simulink model "equalizer_eml"  (Simulink 6.0)
settings: Solver=FixedStepDiscrete  SolverMode=SingleTasking  StartTime=0.0  StopTime=0.1  RelTol=1e-3
InitFcn:
  | equalizer_eml_init
values from neighbouring files (symbols this model uses):
  params = p    [wlan80211a_settings.m]
undefined symbols (not defined in the file or in its folder): qammod, slcm
libraries: commsink2 x4, dspsigattribs x4, commchan2 x2, commdigbbndam2 x2, dsparch4 x1, commrandsrc2 x1, dspsnks4 x1, simulink x1
CloseFcn:
  | clear params
  | clear logsOut
settings Model: CovMetricSettings=dmw  Creator=The Mathworks Inc.  LastModifiedBy=mclark  ExtModeAutoUpdateStatusClock=off
settings DataIOCC: LimitDataPoints=off  SaveOutput=off  SaveTime=off  SignalLoggingName=logsOut
settings OptimizationCC: InlineInvariantSignals=off  LifeSpan=1
settings DebuggingCC: CheckExecutionContextPreStartOutputMsg=on  CheckExecutionContextRuntimeOutputMsg=on  SolverPrmCheckMsg=none
settings HardwareCC: TargetUnknown=on
settings ModelReferenceCC: UpdateModelReferenceTargets=IfOutOfDate
settings RTWCC: SystemTargetFile=ert.tlc  TemplateMakefile=ert_default_tmf  GenerateReport=on  ProcessScript=ert_make_rtw_hook  LaunchReport=on
settings CodeAppCC: IgnoreCustomStorageClasses=off  MangleLength=5
settings ERTTargetCC: TargetFcnLib=ansi_tfl_tmw.mat  GenFloatMathFcnCalls=ANSI_C  GenerateSampleERTMain=on  SupportContinuousTime=on  SupportNonInlinedSFcns=on  RootIOFormat=Individual Arguments  ERTCustomFileTemplate=example_file_process.tlc  InitialValueSource=Model
settings SFSimCC: SFSimApplyToAllLibs=on  SFSimBuildMode=Incremental

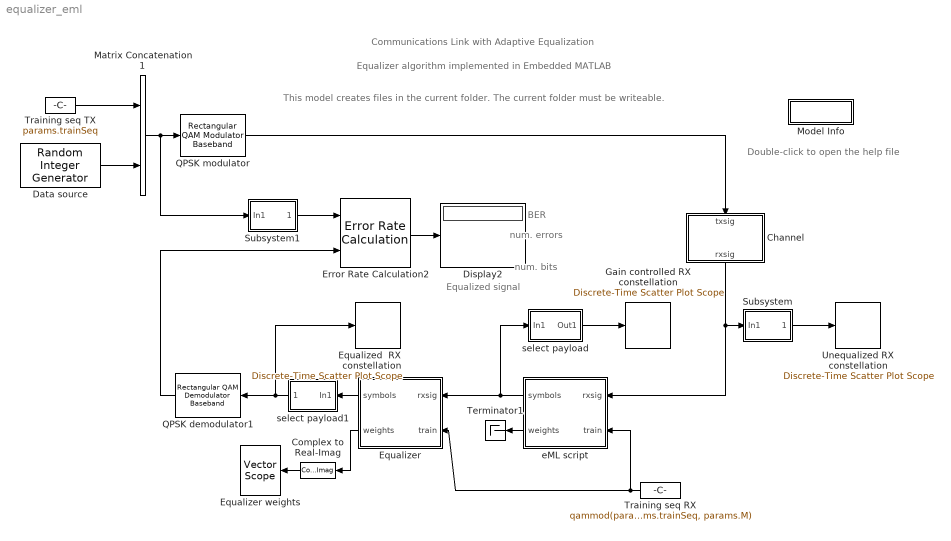
== system equalizer_eml ==
  note: Communications Link with Adaptive Equalization
  note: Equalizer algorithm implemented in Embedded MATLAB
  note: BER
  note: Equalized signal
  note: num. errors
  note: Double-click to open
      | the help file
  note: This model creates files in the current folder.
      | The current folder must be writeable.
  note: num. bits
  " Gain controlled RX constellation" : commsink2/Discrete-Time Scatter Plot Scope  Tag=ScatterPlot  sampPerSymb=1  offsetEye=0  numTraces=200  numNewFrames=100  LineMarkers=.  LineColors=b  fading=on  render=on  AxisGrid=on  xMin=-1.84900078842742  xMax=1.93655728027381  yMin=-1.87362349123512  yMax=1.91193457746611  inphaseLabel=In-phase Amplitude  quadratureLabel=Quadrature Amplitude  openScopeAtSimStart=on  FrameNumber=off  FigPos=[256 31 242 242]  figTitle=''  numLinesMax=8  block_type_=scatter
  Channel : Subsystem  Orientation=down  PropExecContextAcrossSSBoundary=on  mask(Multipath Rician fading chanel){gain_fade=[0 -9], gain_spec=[-10 -60], doppler=0.0001/params.symbolPeriod, SNRdB=60, T=params.symbolPeriod}
      mask prompts: gain_fade "Fading component gains (dB):"; gain_spec "Specular component gains (dB):"; doppler "Maximum Doppler shift (Hz):"; SNRdB "SNR (dB):"; T "Symbol period (s):"
      mask init:
      | gSpec = sum(10.^(gain_spec/10));
      | gFade = sum(10.^(gain_fade)/10);
      | gainChan = sqrt(0.5/(gSpec+gFade));
      | % factor of 0.5 for QPSK
      mask Display: disp('Rician Fading\nChannel')
  Complex to Real-Imag : ComplexToRealImag  Orientation=left  Output=Real
  Data source : commrandsrc2/Random Integer Generator  mul=4  seed=37  Ts=params.sourcePeriod  frameBased=on  sampPerFrame=params.Nsource  orient=off
  Display2 : Display
  Equalized  RX constellation : commsink2/Discrete-Time Scatter Plot Scope  Tag=ScatterPlot  sampPerSymb=1  offsetEye=0  numTraces=200  numNewFrames=100  LineMarkers=.  LineColors=b  fading=on  render=on  AxisGrid=on  xMin=-1.84900078842742  xMax=1.93655728027381  yMin=-1.87362349123512  yMax=1.91193457746611  inphaseLabel=In-phase Amplitude  quadratureLabel=Quadrature Amplitude  openScopeAtSimStart=on  FrameNumber=off  FigPos=[505 31 242 242]  figTitle=''  numLinesMax=8  block_type_=scatter
  Equalizer : Subsystem  Orientation=left  PropExecContextAcrossSSBoundary=on  mask(Receiver processing (adaptive equalizer)){eqMode=RLS, numWeights=6, refTap=4, resetWeights=off}
      mask prompts: eqMode "Adaptive algorithm:"; numWeights "Number of weights:"; refTap "Reference tap:"; resetWeights "Reset weights each frame"
      mask init:
      | if refTap<1 || refTap>numWeights
      | 	error(['Reference tap must be between 1 and ' num2str(numWeights)]);
      | end
      | stepSize = 0.025; % step size
      | lambda = 0.99; % forget factor
      | delta1 = 0.1 + 0i; % diagonal element of inv. corr. mtx.
      mask StyleString: popup(LMS|RLS),edit,edit,checkbox
  Equalizer weights : dspsnks4/Vector Scope  Orientation=left  ScopeProperties=off  Domain=User-defined  HorizSpan=1  DisplayProperties=off  AxisGrid=on  Memory=off  FrameNumber=off  AxisLegend=off  AxisZoom=off  OpenScopeAtSimStart=on  OpenScopeImmediately=off  FigPos=[756 30 251 243]  AxisProperties=off  XUnits=Hertz  XRange=[0...Fs/2]  InheritXIncr=off  XIncr=1  XLabel=delay  YUnits=dB  YLabel=Amplitude  LineProperties=off  LineMarkers=.  LineColors=[0 0 1]
      settings: YMin=-2  YMax=2
  Error Rate Calculation2 : commsink2/Error Rate Calculation  N=0  st_delay=0  cp_mode=Entire frame  subframe=[]  PMode=Port  WsName=ErrorVec  RsMode2=off  stop=off  numErr=100  maxBits=1e6
  Matrix Concatenation1 : simulink/Math Operations/Matrix Concatenation  numInports=2  catMethod=Vertical
  Model Info : Subsystem  LoadFcn=slcm LoadBlock;  InitFcn=slcm('UpdateAllCMBlocksInThisModelInit')  PropExecContextAcrossSSBoundary=on  mask(CMBlock){InitialSaveTempField=, InitialBlockCM=None, BlockCM=None, Frame=on, SaveTempField=, DisplayStringWithTags=Info, MaskDisplayString=Info, HorizontalTextAlignment=Center, LeftAlignmentValue=0.5, SourceBlockDiagram=equalizer_eml, TagMaxNumber=20, CMTag1=, CMTag2=, CMTag3=, CMTag4=, CMTag5=, CMTag6=, CMTag7=, CMTag8=, CMTag9=, CMTag10=, CMTag11=, CMTag12=, CMTag13=, CMTag14=, CMTag15=, CMTag16=, CMTag17=, CMTag18=, CMTag19=, CMTag20=}
      mask help: This block allows revision control information to be displayed within the model.
      settings: CopyFcn=slcm CopyBlock;  DeleteFcn=slcm Cancel;  PostSaveFcn=slcm('UpdateAllCMBlocksInThisModel')  NameChangeFcn=slcm Rename;  OpenFcn=commdemohelp;
      mask Display: text(str2num(LeftAlignmentValue), 0.5, MaskDisplayString, 'HorizontalAlignment', HorizontalTextAlignment)
  QPSK demodulator1 : commdigbbndam2/Rectangular QAM Demodulator Baseband  Orientation=left  M=params.M  OutType=Integer  Dec=Binary  PowType=Min. distance between symbols  MinDist=2  AvgPow=1  PeakPow=1  Ph=0  numSamp=1
  QPSK modulator : commdigbbndam2/Rectangular QAM Modulator Baseband  M=params.M  InType=Integer  Enc=Binary  PowType=Min. distance between symbols  MinDist=2  AvgPow=1  PeakPow=1  Ph=0  numSamp=1
  Subsystem : Subsystem  PropExecContextAcrossSSBoundary=on
      mask Display: disp('Select\nPayload')
  Subsystem1 : Subsystem  PropExecContextAcrossSSBoundary=on
      mask Display: disp('Select\nPayload')
  Terminator1 : Terminator
  Training seq RX : Constant  Orientation=left  Value=qammod(params.trainSeq, params.M)
  Training seq TX : Constant  Value=params.trainSeq
  Unequalized RX constellation : commsink2/Discrete-Time Scatter Plot Scope  Tag=ScatterPlot  sampPerSymb=1  offsetEye=0  numTraces=500  numNewFrames=50  LineMarkers=.  LineColors=b  fading=on  render=on  AxisGrid=on  xMin=-2  xMax=2  yMin=-2  yMax=2  inphaseLabel=In-phase Amplitude  quadratureLabel=Quadrature Amplitude  openScopeAtSimStart=on  FrameNumber=off  FigPos=[7 31 242 243]  figTitle=''  numLinesMax=8  block_type_=scatter
  eML script : Stateflow chart  Orientation=left  PropExecContextAcrossSSBoundary=on
  select payload : Subsystem  PropExecContextAcrossSSBoundary=on
      mask Display: disp('Select\nPayload')
  select payload1 : Subsystem  Orientation=left  PropExecContextAcrossSSBoundary=on
      mask Display: disp('Select\nPayload')
  wires:
  Subsystem/1(Out1) -> Unequalized RX constellation/1
  eML script/2(weights) -> Terminator1/1
  Training seq TX/1 -> Matrix Concatenation1/1
  Data source/1 -> Matrix Concatenation1/2
  Matrix Concatenation1/1 -> QPSK modulator/1, Subsystem1/1(In1)
  QPSK modulator/1 -> Channel/1(txsig)
  Subsystem1/1(Out1) -> Error Rate Calculation2/1
  Error Rate Calculation2/1 -> Display2/1
  eML script/1(symbols) -> select payload/1(In1), Equalizer/1(rxsig)
  select payload/1(Out1) -> " Gain controlled RX constellation"/1
  Channel/1(rxsig) -> eML script/1(rxsig), Subsystem/1(In1)
  Training seq RX/1 -> eML script/2(train), Equalizer/2(train)
  Equalizer/1(symbols) -> select payload1/1(In1)
  select payload1/1(Out1) -> QPSK demodulator1/1, Equalized  RX constellation/1
  QPSK demodulator1/1 -> Error Rate Calculation2/2
  Equalizer/2(weights) -> Complex to Real-Imag/1
  Complex to Real-Imag/1 -> Equalizer weights/1

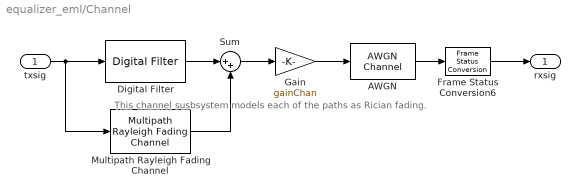
== system equalizer_eml/Channel ==
  note: This channel susbsystem models each
      | of the paths as Rician fading.
  txsig : Inport  LatchInput=off
  AWGN : commchan2/AWGN Channel  seed=67  noiseMode="Signal to noise ratio  (SNR)"  EbNodB=10  EsNodB=10  SNRdB=SNRdB  bitsPerSym=1  Ps=1  Tsym=1  variance=1
  Digital Filter : dsparch4/Digital Filter  DialogController=dspDDGCreate  DialogControllerArgs=DataTag0  TypePopup=FIR (all zeros)  IIRFiltStruct=Direct form II transposed  AllPoleFiltStruct=Direct form  FIRFiltStruct=Direct form  CoeffSource=Specify via dialog  NumCoeffs=10.^(gain_spec/20)  DenCoeffs=[1 0.1]  BiQuadCoeffs=[1 0.3 0.4 1 0.1 0.2]  LatticeCoeffs=[0.2 0.4]  denIgnore=on  FiltPerSampPopup=One filter per frame  IC=0  ICnum=0  ICden=0  roundingMode=Floor  overflowMode=off  ScaleValues=1  scaleValueFracLength=14  stageInFracLength=15  stageOutFracLength=15
  Frame Status Conversion6 : dspsigattribs/Frame Status Conversion  growRefPort=off  outframe=Sample-based
  Gain : Gain  Gain=gainChan  SaturateOnIntegerOverflow=on
  Multipath Rayleigh Fading Channel : commchan2/Multipath Rayleigh Fading Channel  Fd=doppler  simTs=T  delayVec=(0:length(gain_fade)-1)*T  gainVecdB=gain_fade  normGain=off  Seed=73
  Sum : Sum  Inputs=|++  SaturateOnIntegerOverflow=on
  rxsig : Outport
  wires:
  AWGN/1 -> Frame Status Conversion6/1
  txsig/1 -> Digital Filter/1, Multipath Rayleigh Fading Channel/1
  Sum/1 -> Gain/1
  Gain/1 -> AWGN/1
  Digital Filter/1 -> Sum/1
  Multipath Rayleigh Fading Channel/1 -> Sum/2
  Frame Status Conversion6/1 -> rxsig/1

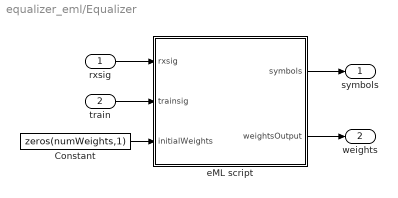
== system equalizer_eml/Equalizer ==
  rxsig : Inport  LatchInput=off
  train : Inport  Port=2  LatchInput=off
  Constant : Constant  Value=zeros(numWeights,1)  VectorParams1D=off
  eML script : Stateflow chart  PropExecContextAcrossSSBoundary=on
  symbols : Outport
  weights : Outport  Port=2
  wires:
  eML script/1(symbols) -> symbols/1
  eML script/2(weightsOutput) -> weights/1
  train/1 -> eML script/2(trainsig)
  rxsig/1 -> eML script/1(rxsig)
  Constant/1 -> eML script/3(initialWeights)

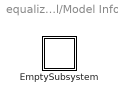
== system equalizer_eml/Model Info ==
  EmptySubsystem : Subsystem  PropExecContextAcrossSSBoundary=on

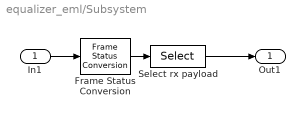
== system equalizer_eml/Subsystem ==
  In1 : Inport  LatchInput=off
  Frame Status Conversion : dspsigattribs/Frame Status Conversion  growRefPort=off  outframe=Frame-based
  Select rx payload : Selector  Elements=(params.Ntrain+1):(params.Nsymbols-10)  InputPortWidth=params.Nsymbols
  Out1 : Outport
  wires:
  In1/1 -> Frame Status Conversion/1
  Select rx payload/1 -> Out1/1
  Frame Status Conversion/1 -> Select rx payload/1

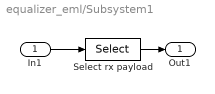
== system equalizer_eml/Subsystem1 ==
  In1 : Inport  LatchInput=off
  Select rx payload : Selector  Elements=(params.Ntrain+1):(params.Nsymbols-10)  InputPortWidth=params.Nsymbols
  Out1 : Outport
  wires:
  In1/1 -> Select rx payload/1
  Select rx payload/1 -> Out1/1

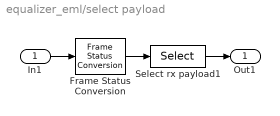
== system equalizer_eml/select payload ==
  In1 : Inport  LatchInput=off
  Frame Status Conversion : dspsigattribs/Frame Status Conversion  growRefPort=off  outframe=Frame-based
  Select rx payload1 : Selector  Elements=(params.Ntrain+1):(params.Nsymbols-10)  InputPortWidth=params.Nsymbols
  Out1 : Outport
  wires:
  Select rx payload1/1 -> Out1/1
  In1/1 -> Frame Status Conversion/1
  Frame Status Conversion/1 -> Select rx payload1/1

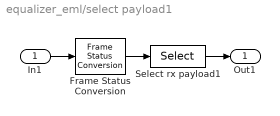
== system equalizer_eml/select payload1 ==
  In1 : Inport  LatchInput=off
  Frame Status Conversion : dspsigattribs/Frame Status Conversion  growRefPort=off  outframe=Frame-based
  Select rx payload1 : Selector  Elements=(params.Ntrain+1):(params.Nsymbols-10)  InputPortWidth=params.Nsymbols
  Out1 : Outport
  wires:
  Frame Status Conversion/1 -> Select rx payload1/1
  In1/1 -> Frame Status Conversion/1
  Select rx payload1/1 -> Out1/1

== system equalizer_eml/Model Info/EmptySubsystem ==

== matlab function eML script ==
  data: rxsig input double; train input double; symbols output double size=size(rxsig); weights output double
function [symbols, weights] = gaincontrol(rxsig, train)
% 1-tap adaptive equalizer using RLS algorithm

% Equalizer settings
lambda = 0.99; % forgetting factor for RLS

% Initialize
Delta = 0.1+0j; % inv. corr. parameter
weights = 0+0j;    

symbols = zeros(length(rxsig),1);
for n = 1:length(rxsig)
    u = rxsig(n);  % received sample
    y = conj(weights) * u;  % output
    if n<=length(train)
        % training mode
        d = train(n);
    else
        % decision-directed mode
        d = detect(real(y)) + 1j*detect(imag(y));
    end
    % Single-tap RLS
    Delta = 1/(lambda/Delta + u*conj(u));
    G = Delta * u;
    e = d - y;  % symbol estimation error
    weights = weights + G*conj(e);  % update weights
    symbols(n) = y;
end


function y = detect(x);
if real(x)<0, y=-1; else y=1; end

== matlab function Equalizer/eML script ==
  data: rxsig input double; trainsig input double; initialWeights input double; symbols output double size=size(rxsig); weightsOutput output double; resetWeights parameter double; eqMode parameter double; refTap parameter double; stepSize parameter double; lambda parameter double; delta1 parameter double
function [symbols, weightsOutput] = equalizer(rxsig, trainsig, initialWeights, resetWeights, eqMode, refTap, stepSize, lambda, delta1)
% Adaptive equalizer using LMS or RLS algorithm

% Equalizer settings
M = length(initialWeights); % number of tap weights

persistent weights
if(isempty(weights))
    weights = initialWeights + 0j;
end

% Initialize
G = zeros(M, 1) + 0j; % Gain vector (both LMS and RLS)
Delta = zeros(M, M) + 0j;  Delta(1:M+1:end) = delta1;  % inv. corr. mtx.
if resetWeights==1
    weights = initialWeights + 0j;   
end
u = zeros(M, 1) + 0j; % input vector (to tap weights)
delay = refTap - 1;
symbols = zeros(length(rxsig),1);
for n = 1:length(rxsig)
    u = [rxsig(n); u(1:M-1)];  % tapped delay line
    if n >= delay
        y = weights' * u;
        m = n - delay + 1;
        if n<=length(trainsig)
            % training mode
            d = trainsig(m);  
        else
            % decision-directed mode
            d = detect(real(y)) + 1j*detect(imag(y));
        end
        e = d - y;  % symbol estimation error
        if eqMode==1
            % LMS
            G = stepSize*u;
        else
            % RLS
            G = Delta * u / (lambda + u'*Delta*u);
            Delta = 1/lambda * (Delta - G*u'*Delta);
        end
        weights = weights + G*conj(e);  % update weights
        symbols(m) = y;	% note: last few symbols not estimated
    end
end
weightsOutput = weights;

function y = detect(x)
if real(x)<0, y=-1; else y=1; end
